simulink model "Wind_turbine_model_L"  (R2020a)
settings: Solver=ode45  StartTime=0.0  StopTime=10  RelTol=1e-3
model workspace (MAT data in the model file):
  Tw = Simulink.Parameter
  Tw.DataType = 'auto'
  Tw.Dimensions = [0 0]
undefined symbols (not defined in the file): a1, a2, a3, a4, a5, a6, a7, a8, Ad, D, denp, dent, DiscIntNeverNeededParam, f, Fs, fsw, J, ki_id, ki_n, Kopt, kp_id, kp_n, Lm, Lr, Ls, Lsi, N, nump, numt, p, Ps, Rr, Rs, sigbuilder_block, sigma, Tem, Tgd_max, Tie, Tiu, Tix, Tpe, Tpu, Tpx, Ts, Vbus, Vs, WT_Params, X, Y, Z
libraries: fl_lib x18, nesl_utility x10, sm_lib x9, powerlib x8, sdl_lib x3, powerlib_meascontrol x1, simulink x1, Yaw_Actuation_Lib x1
settings Model: Creator=param  LastModifiedBy=param

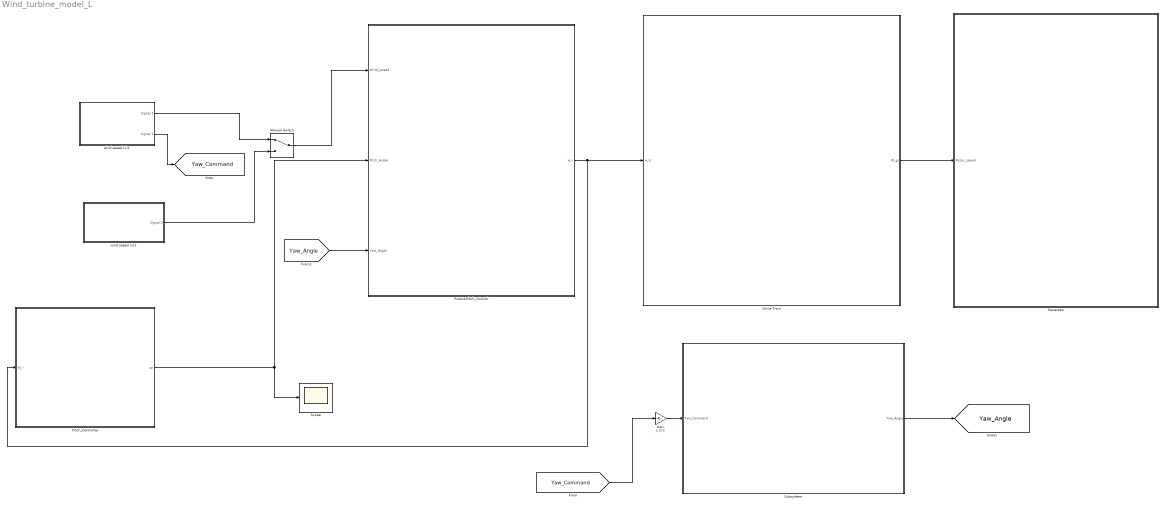
== system Wind_turbine_model_L ==
  Drive Train : Subsystem
  Gain : Gain  Gain=0.075
  Generator : Subsystem
  Manual Switch : ManualSwitch
  Pitch_Controller : Subsystem
  Rotor&Pitch_Control : Subsystem
  Scope : Scope
  Subsystem : Subsystem
  wind speed (v)1 : Subsystem  Tag=STV Subsys  LoadFcn=sigbuilder_block('load');  StartFcn=sigbuilder_block('start');  StopFcn=sigbuilder_block('stop');  ClipboardFcn=sigbuilder_block('clipboard');  mask(Sigbuilder block){tuvar=[0:10]}
      mask help: Simulink:masks:SigbuilderBlock_MD
      mask init:
      | if ~strcmp(get_param(bdroot(gcbh),'SimulationStatus'),'stopped') tuvar = sigbuilder_block('maskInit'); end
      settings: CopyFcn=sigbuilder_block('copy');  DeleteFcn=sigbuilder_block('delete');  ModelCloseFcn=sigbuilder_block('modelClose');  PreSaveFcn=sigbuilder_block('preSave');  PauseFcn=sigbuilder_block('pause');  ContinueFcn=sigbuilder_block('continue');  NameChangeFcn=sigbuilder_block('namechange');  OpenFcn=sigbuilder_block('open',[6 0 1012.5 477.75 ]);  CloseFcn=sigbuilder_block('close');
      mask Display: plot(0, 0, 100, 100,[2, 2, 32, 32, 2], [68, 8, 8, 68, 68],[32, 2], [38, 38], [32, 19, 2],[53, 60, 44], [32, 17, 17, 2],[16, 16, 31, 31]);txt = getActiveGroup(gcbh);text(2, 100, txt,'verticalAlignment', 'top');
  wind speed (v)2 : Subsystem  Tag=STV Subsys  LoadFcn=sigbuilder_block('load');  StartFcn=sigbuilder_block('start');  StopFcn=sigbuilder_block('stop');  ClipboardFcn=sigbuilder_block('clipboard');  mask(Sigbuilder block){tuvar=[0:10]}
      mask help: Simulink:masks:SigbuilderBlock_MD
      mask init:
      | if ~strcmp(get_param(bdroot(gcbh),'SimulationStatus'),'stopped') tuvar = sigbuilder_block('maskInit'); end
      settings: CopyFcn=sigbuilder_block('copy');  DeleteFcn=sigbuilder_block('delete');  ModelCloseFcn=sigbuilder_block('modelClose');  PreSaveFcn=sigbuilder_block('preSave');  PauseFcn=sigbuilder_block('pause');  ContinueFcn=sigbuilder_block('continue');  NameChangeFcn=sigbuilder_block('namechange');  OpenFcn=sigbuilder_block('open',[289.8 114 442.2 307.8 ]);  CloseFcn=sigbuilder_block('close');
      mask Display: plot(0, 0, 100, 100,[2, 2, 32, 32, 2], [68, 8, 8, 68, 68],[32, 2], [38, 38], [32, 19, 2],[53, 60, 44], [32, 17, 17, 2],[16, 16, 31, 31]);txt = getActiveGroup(gcbh);text(2, 100, txt,'verticalAlignment', 'top');
  tag scope: Yaw_Angle=global, Yaw_Command=global
  wires:
  Drive Train/1(W_gr) -> Generator/1(Rotor_speed)
  Rotor&Pitch_Control/1(w_r) -> Drive Train/1(w_tr), Pitch_Controller/1(W_r)
  Pitch_Controller/1(up) -> Scope/1, Rotor&Pitch_Control/2(Pitch_Angle)
  wind speed (v)2/1(Signal 2) -> Manual Switch/2
  Manual Switch/1 -> Rotor&Pitch_Control/1(Wind_Speed)
  wind speed (v)1/1(Signal 2) -> Manual Switch/1
  wind speed (v)1/2(Signal 1) -> [Yaw_Command]
  [Yaw_Command] -> Gain/1
  Subsystem/1(Yaw_Angle) -> [Yaw_Angle]
  [Yaw_Angle] -> Rotor&Pitch_Control/3(Yaw_Angle)
  Gain/1 -> Subsystem/1(Yaw_Command)

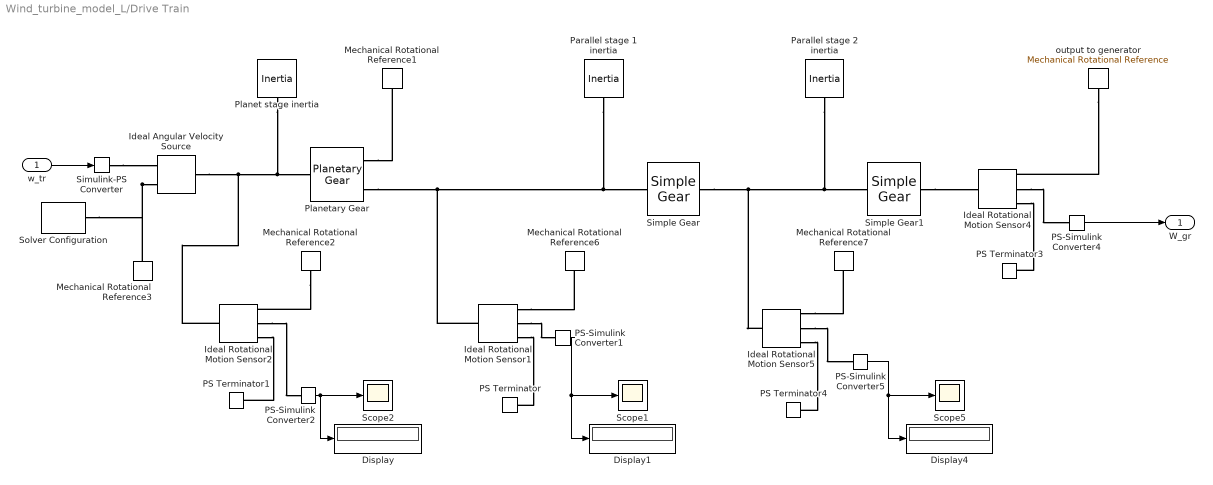
== system Wind_turbine_model_L/Drive Train ==
  w_tr : Inport
  Display : Display
  Display1 : Display
  Display4 : Display
  Ideal Angular Velocity Source : fl_lib/Mechanical/Mechanical Sources/Ideal Angular Velocity Source
  Ideal Rotational Motion Sensor{1..2,4..5} (4 alike) : fl_lib/Mechanical/Mechanical Sensors/Ideal Rotational Motion Sensor  wrap_angle=simscape.enum.onoff.off  offset=0 rad
  Mechanical Rotational Reference{1..3,6..7} (5 alike) : fl_lib/Mechanical/Rotational Elements/Mechanical Rotational Reference
  PS Terminator{,1,3..4} (4 alike) : fl_lib/Physical Signals/Sinks/PS Terminator
  PS-Simulink Converter{1..2,4..5} (4 alike) : nesl_utility/PS-Simulink Converter  PhysicalDomain=network_engine_domain  SubClassName=ps_output  LeftPortType=input  RightPortType=output  PseudoPeriodic=off  Frequencies=[]  Unit=inherit  AffineConversion=off
  Parallel stage 1 inertia : fl_lib/Mechanical/Rotational Elements/Inertia  inertia=100 kg*m^2  w_specify=off  w_priority=High  w=0 rad/s  w_nominal_specify=off  w_nominal_unit=rad/s  w_nominal_value=1  t_specify=off  t_priority=None  t=0 N*m  t_nominal_specify=off  t_nominal_unit=N*m  t_nominal_value=1
  Parallel stage 2 inertia : fl_lib/Mechanical/Rotational Elements/Inertia  inertia=100 kg*m^2  w_specify=off  w_priority=High  w=0 rad/s  w_nominal_specify=off  w_nominal_unit=rad/s  w_nominal_value=1  t_specify=off  t_priority=None  t=0 N*m  t_nominal_specify=off  t_nominal_unit=N*m  t_nominal_value=1
  Planet stage inertia : fl_lib/Mechanical/Rotational Elements/Inertia  inertia=100 kg*m^2  w_specify=off  w_priority=High  w=0 rad/s  w_nominal_specify=off  w_nominal_unit=rad/s  w_nominal_value=1  t_specify=off  t_priority=None  t=0 N*m  t_nominal_specify=off  t_nominal_unit=N*m  t_nominal_value=1
  Planetary Gear : sdl_lib/Gears/Planetary Gear  rs_ratio=7  friction_model=sdl.enum.gear_friction.none  mu_visc=[0, 0] N*m/(rad/s)  efficiency=[.96, .98]  temperature_TLU=[280, 300, 320] K  efficiency_sp_TLU=[.95, .9, .85]  efficiency_rp_TLU=[.95, .9, .85]  pwr_thr=[.001, .001] W  thermal_mass=50 J/K  T_init=300 K  model_inertia=simscape.enum.onoff.off  planet_inertia=100 kg*m^2
      settings: SourceProductBaseCode=LD
  Scope1 : Scope
  Scope2 : Scope
  Scope5 : Scope
  Simple Gear : sdl_lib/Gears/Simple Gear  ratio=1/4.5  rotation_direction=2  friction_model=sdl.enum.gear_efficiencies_load.off  T_noload=0.1 N*m  T_nom=5 N*m  efficiency_nom=0.8  efficiency=0.8  mu_visc=[0, 0] N*m/(rad/s)  w_thr=0.01 rad/s  pwr_thr=0.001 W  enable_faults=simscape.enum.onoff.off  efficiency_fault=0.05  external_fault=simscape.enum.onoff.off  temporal_fault=simscape.enum.onoff.off  fault_time=5 s  fault_angles=pi / 12 rad  report_fault=1  temperature_TLU=[280, 300, 320] K  load_TLU=[1, 5, 10] N*m  efficiency_TLU=[.95, .9, .85]  efficiency_TLU2=[.85, .8, .75; .95, .9, .85; .85, .8, .7]  thermal_mass=50 J/K  T_init=300 K
  Simple Gear1 : sdl_lib/Gears/Simple Gear  ratio=1/3.15  rotation_direction=2  friction_model=sdl.enum.gear_efficiencies_load.off  T_noload=0.1 N*m  T_nom=5 N*m  efficiency_nom=0.8  efficiency=0.8  mu_visc=[0, 0] N*m/(rad/s)  w_thr=0.01 rad/s  pwr_thr=0.001 W  enable_faults=simscape.enum.onoff.off  efficiency_fault=0.05  external_fault=simscape.enum.onoff.off  temporal_fault=simscape.enum.onoff.off  fault_time=5 s  fault_angles=pi / 12 rad  report_fault=1  temperature_TLU=[280, 300, 320] K  load_TLU=[1, 5, 10] N*m  efficiency_TLU=[.95, .9, .85]  efficiency_TLU2=[.85, .8, .75; .95, .9, .85; .85, .8, .7]  thermal_mass=50 J/K  T_init=300 K
  Simulink-PS Converter : nesl_utility/Simulink-PS Converter  PhysicalDomain=network_engine_domain  SubClassName=ps_input  LeftPortType=input  RightPortType=output  PseudoPeriodic=off  Frequencies=[]  NoiseDistribution=none  NoiseParameters=[]  Unit=1  AffineConversion=off  FilteringAndDerivatives=filter  SimscapeFilterOrder=2  InputFilterTimeConstant=0.001  UdotUserProvided=0
  Solver Configuration : nesl_utility/Solver Configuration  PhysicalDomain=network_engine_domain  SubClassName=solver  LeftPortType=input  RightPortType=generic  Tones=[]  Harmonics=[]  SimulateNoise=off  Profile=off  UseLocalSampling=off  EnableSwitchedLinearOptims=on  FrequencyDomain=off  UseCCode=off  RelTol=0.001  AbsTol=1e-06  MinStep=1e-09  ToWorkspace=off  RevertToSquareIcSolve=off  NumHomotopyIterations=100  PhasorMode=off  PhasorModeNumHarmonics=1  DoDC=off  ResidualTolerance=1e-09  UseLocalSolver=off  LocalSolverChoice=NE_BACKWARD_EULER_ADVANCER  LocalSolverSampleTime=0.001  DoFixedCost=off  MaxNonlinIter=3  MaxModeIter=2  LinearAlgebra=auto  EquationFormulation=NE_TIME_EF  DelaysMemoryBudget=1024  AutomaticFiltering=on  FilteringTimeConstant=0.001  PartitionStorageMethod=AS_NEEDED  PartitionMemoryBudget=1024  PartitionMethod=ROBUST
  output to generator : fl_lib/Mechanical/Rotational Elements/Mechanical Rotational Reference
  W_gr : Outport
  wires:
  PS-Simulink Converter1/1 -> Scope1/1, Display1/1
  PS-Simulink Converter2/1 -> Display/1, Scope2/1
  PS-Simulink Converter5/1 -> Display4/1, Scope5/1
  PS-Simulink Converter4/1 -> W_gr/1
  w_tr/1 -> Simulink-PS Converter/1
  connections:
  Ideal Angular Velocity Source/LConn1 -- Ideal Rotational Motion Sensor2/LConn1 -- Planet stage inertia/LConn1 -- Planetary Gear/LConn1
  Planetary Gear/RConn1 -- Mechanical Rotational Reference1/LConn1
  Ideal Angular Velocity Source/RConn2 -- Mechanical Rotational Reference3/LConn1 -- Solver Configuration/RConn1
  Ideal Rotational Motion Sensor1/RConn2 -- PS-Simulink Converter1/LConn1
  Ideal Rotational Motion Sensor5/RConn3 -- PS Terminator4/LConn1
  Planetary Gear/RConn2 -- Ideal Rotational Motion Sensor1/LConn1 -- Simple Gear/LConn1 -- Parallel stage 1 inertia/LConn1
  Ideal Rotational Motion Sensor1/RConn1 -- Mechanical Rotational Reference6/LConn1
  Mechanical Rotational Reference2/LConn1 -- Ideal Rotational Motion Sensor2/RConn1
  Ideal Rotational Motion Sensor4/RConn2 -- PS-Simulink Converter4/LConn1
  Ideal Rotational Motion Sensor5/RConn2 -- PS-Simulink Converter5/LConn1
  Ideal Rotational Motion Sensor2/RConn3 -- PS Terminator1/LConn1
  Simple Gear1/RConn1 -- Ideal Rotational Motion Sensor4/LConn1
  Simple Gear/RConn1 -- Ideal Rotational Motion Sensor5/LConn1 -- Parallel stage 2 inertia/LConn1 -- Simple Gear1/LConn1
  Ideal Rotational Motion Sensor4/RConn3 -- PS Terminator3/LConn1
  Ideal Rotational Motion Sensor5/RConn1 -- Mechanical Rotational Reference7/LConn1
  Ideal Rotational Motion Sensor2/RConn2 -- PS-Simulink Converter2/LConn1
  output to generator/LConn1 -- Ideal Rotational Motion Sensor4/RConn1
  Ideal Rotational Motion Sensor1/RConn3 -- PS Terminator/LConn1
  Simulink-PS Converter/RConn1 -- Ideal Angular Velocity Source/RConn1

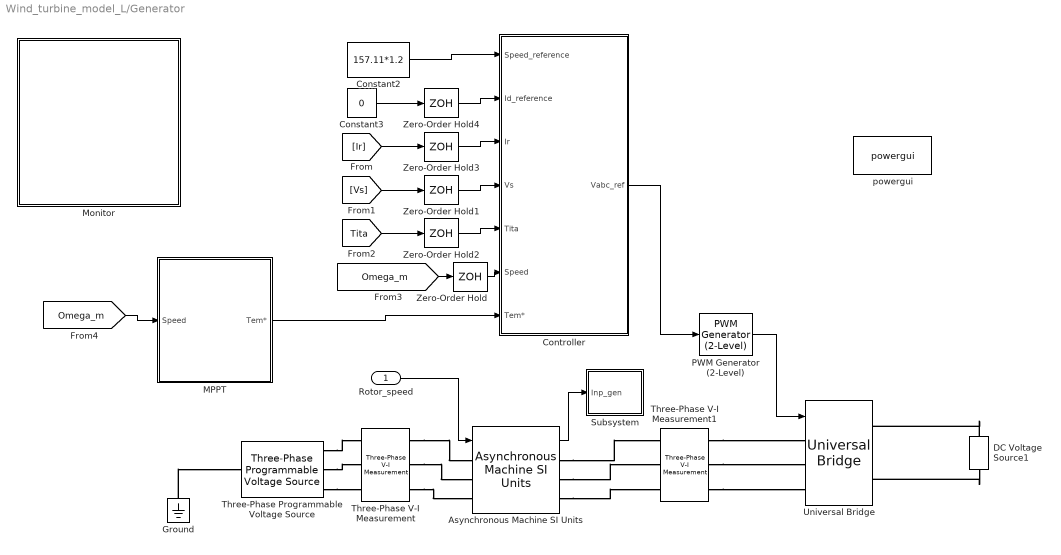
== system Wind_turbine_model_L/Generator ==
  Rotor_speed : Inport
  Asynchronous Machine SI Units : powerlib/Machines/Asynchronous Machine SI Units  RotorType=Wound  PresetModel=No  MechanicalLoad=Speed w  ShowDetailedParameters=on  ReferenceFrame=Rotor  Units=SI  MeasurementBus=off  NominalParameters=[Ps Vs f]  Stator=[Rs, Lsi]  Rotor=[Rr, Lsi]  Cage1=[0.4155 0.002066]  Cage2=[0.4168 0.0003495]  Lm=Lm  Mechanical=[J D 2]  PolePairs=2  InitialConditions=[1 0 0 0 0 0 0 0]  SimulateSaturation=off  Saturation=[14.03593122, 27.81365428, 53.79336849, 72.68890987, 97.98006896, 148.6815601, 215.7428561, 302.9841135, 428.7778367 ; 230, 322, 414, 460, 506, 552, 598, 644, 690]  LoadFlowParameters=1492000  TsPowergui=0  TsBlock=-1  IterativeModel=Trapezoidal non iterative  IterativeDiscreteModel=Trapezoidal non iterative  Pmec=1.492e+006
  Constant2 : Constant  Value=157.11*1.2
  Constant3 : Constant  Value=0
  Controller : Subsystem
  DC Voltage Source1 : powerlib/Electrical Sources/DC Voltage Source  Amplitude=Vbus  Measurements=None
  Ground : powerlib/Elements/Ground  LConnTagsString=a
  MPPT : Subsystem
  Monitor : Subsystem
  PWM Generator (2-Level) : powerlib_meascontrol/Pulse & Signal Generators/PWM Generator (2-Level)  ModulatorType=Three-phase bridge (6 pulses)  ModulatorMode=Unsynchronized  Fc=fsw  Pc=90  nF=27  MinMax="[ -1  1 ]"  SamplingTechnique=Symmetrical regular (single edge)  ModulatingSignals=off  m=0.8  Freq=60  Phase=0  Ts=0  ShowCarrierOutport=off
  Subsystem : Subsystem
  Three-Phase Programmable Voltage Source : powerlib/Electrical Sources/Three-Phase Programmable Voltage Source  PositiveSequence=[Vs 0 f]  VariationEntity=None  VariationType=Table of time-amplitude pairs  VariationTypeAlt=Step  VariationStep=0.5  VariationRate=10  VariationMagnitude=0.3  VariationFrequency=2  VariationTiming=[1 2]  VariationPhaseA=off  Amplitudes=[1 0.8 1.2 1.0]  TimeValues=[0 0.1 0.15 0.2]  HarmonicGeneration=off  HarmonicA=[3 0.2 -25 0]  HarmonicB=[2 0.15 35 2]  Timing="[0.05  3]"  BusType=swing  Pref=0  Qref=0  Qmin=-inf  Qmax=inf
  Three-Phase V-I Measurement : powerlib/Measurements/Three-Phase V-I Measurement  VoltageMeasurement=phase-to-ground  SetLabelV=on  LabelV=Vs  Vpu=on  VpuLL=off  CurrentMeasurement=yes  SetLabelI=on  LabelI=Is  Ipu=off  Pbase=100e6  Vbase=500e3  OutputType=Complex  PhasorSimulation=off  PSBequivalent=0
  Three-Phase V-I Measurement1 : powerlib/Measurements/Three-Phase V-I Measurement  VoltageMeasurement=no  SetLabelV=off  LabelV=Vr  Vpu=off  VpuLL=off  CurrentMeasurement=yes  SetLabelI=on  LabelI=Ir  Ipu=off  Pbase=100e6  Vbase=500e3  OutputType=Complex  PhasorSimulation=off  PSBequivalent=0
  Universal Bridge : powerlib/Power Electronics/Universal Bridge  Arms=3  SnubberResistance=1e5  SnubberCapacitance=inf  Device=Ideal Switches  Ron=1e-3  Lon=0  ForwardVoltages="[  0  0  ]"  ForwardVoltage=0  GTOparameters=[ 10e-6 , 20e-6 ]  IGBTparameters=[ 1e-6 , 2e-6 ]  Measurements=None  Measurements_2=None  converterType=Rectifier
  Zero-Order Hold{,1..4} (5 alike) : ZeroOrderHold  SampleTime=1/fsw
  powergui : powerlib/powergui  Priority=1  SimulationMode=Discrete  SampleTime=Ts  frequency=60  Iterations=50  frequencyindice=50  Pbase=100e6  ErrMax=1e-4  UnitsV=kV  UnitsW=MW  buscounter=0  FunctionMessages=off  echomessages=off  EnableUseOfTLC=off  CurrentSourceSwitches=off  DisableSnubberDevices=off  DisableRonSwitches=off  DisableVfSwitches=off  DisplayEquations=off  AutomaticDiscreteSolvers=off  SolverType=Tustin/Backward Euler (TBE)  Interpol=off  ExternalGateDelay=off  methode=off  Ts=100  x0status=blocks  SPID=on  SwTol=0  HookPort=off  NonlinearTolerance=1e-4  nMaxIteration=100  ContinueOnMaxIteration=off  RestoreLinks=warning  ResistiveCurrentMeasurement=off  Frange=[0:2:500]  Ylog=off  Xlog=on  ShowGrid=off  save=off  variable=ZData  structure=0  ZoomFFT=off  StartTime=0.0  cycles=1  DisplayStyle=1  fundamental=60  FreqAxis=off  MaxFrequency=1000  frequencyindicesteady=1  RmsSteady=1  display=off
  wires:
  Zero-Order Hold2/1 -> Controller/5(Tita)
  [Tita] -> Zero-Order Hold2/1
  Zero-Order Hold/1 -> Controller/6(Speed)
  [Vs] -> Zero-Order Hold1/1
  Zero-Order Hold4/1 -> Controller/2(Id_reference)
  Zero-Order Hold1/1 -> Controller/4(Vs)
  [Ir] -> Zero-Order Hold3/1
  Asynchronous Machine SI Units/1 -> Subsystem/1(Inp_gen)
  PWM Generator (2-Level)/1 -> Universal Bridge/1
  Constant2/1 -> Controller/1(Speed_reference)
  Constant3/1 -> Zero-Order Hold4/1
  [Omega_m] -> Zero-Order Hold/1
  Zero-Order Hold3/1 -> Controller/3(Ir)
  Controller/1(Vabc_ref) -> PWM Generator (2-Level)/1
  Rotor_speed/1 -> Asynchronous Machine SI Units/1
  [Omega_m] -> MPPT/1(Speed)
  MPPT/1(Tem*) -> Controller/7(Tem*)
  connections:
  Three-Phase V-I Measurement1/LConn3 -- Universal Bridge/LConn3
  Asynchronous Machine SI Units/RConn1 -- Three-Phase V-I Measurement1/RConn1
  Three-Phase V-I Measurement/RConn1 -- Asynchronous Machine SI Units/LConn1
  DC Voltage Source1/LConn1 -- Universal Bridge/RConn2
  Three-Phase Programmable Voltage Source/RConn3 -- Three-Phase V-I Measurement/LConn3
  Three-Phase V-I Measurement1/LConn2 -- Universal Bridge/LConn2
  Three-Phase Programmable Voltage Source/RConn2 -- Three-Phase V-I Measurement/LConn2
  Three-Phase Programmable Voltage Source/RConn1 -- Three-Phase V-I Measurement/LConn1
  Three-Phase V-I Measurement1/LConn1 -- Universal Bridge/LConn1
  Three-Phase V-I Measurement/RConn2 -- Asynchronous Machine SI Units/LConn2
  Three-Phase V-I Measurement/RConn3 -- Asynchronous Machine SI Units/LConn3
  Asynchronous Machine SI Units/RConn3 -- Three-Phase V-I Measurement1/RConn3
  Ground/LConn1 -- Three-Phase Programmable Voltage Source/LConn1
  DC Voltage Source1/RConn1 -- Universal Bridge/RConn1
  Asynchronous Machine SI Units/RConn2 -- Three-Phase V-I Measurement1/RConn2

== system Wind_turbine_model_L/Pitch_Controller ==
  note: um
  note: Wref
  W_r : Inport
  Controller : Subsystem
  Reference : TransferFcn  Denominator=[1 1]
  Step : Step  Time=0  After=1.8  SampleTime=0
  Sum3 : Sum  Inputs=|+-
  up : Outport
  wires:
  W_r/1 -> Sum3/2
  Step/1 -> Controller/2(um), Reference/1
  Reference/1 -> Sum3/1, Controller/1(xm)
  Sum3/1 -> Controller/3(ey)
  Controller/1(up) -> up/1

== system Wind_turbine_model_L/Rotor&Pitch_Control ==
  Wind_Speed : Inport
  Pitch_Angle : Inport  Port=2
  Yaw_Angle : Inport  Port=3
  Abs : Abs
  Constant : Constant  Commented=on  Value=Tgd_max
  Wr Plant : Subsystem
  w_r : Outport
  wires:
  Wr Plant/1(Wr(s)) -> w_r/1
  Wind_Speed/1 -> Wr Plant/1(v(s))
  [Tem_ref] -> Abs/1
  Abs/1 -> Wr Plant/3(Tgd(s))
  Pitch_Angle/1 -> Wr Plant/2(Betad(s))
  Yaw_Angle/1 -> Wr Plant/4(Yaw_Angle)

== system Wind_turbine_model_L/Subsystem ==
  Yaw_Command : Inport
  PID Controller : simulink/Continuous/PID Controller  Controller=PID  Form=Parallel  TimeDomain=Continuous-time  UseExternalTs=off  SampleTime=-1  IntegratorMethod=Forward Euler  FilterMethod=Forward Euler  ControllerParametersSource=internal  P=2.88422427280199  I=9.43357368987043  D=0.0596373379151778  UseFilter=on  N=693.993801659791  TunerSelectOption=Transfer Function Based (PID Tuner App)  InitialConditionSource=internal  InitialConditionForIntegrator=0  InitialConditionForFilter=0  DifferentiatorICPrevScaledInput=0  ExternalReset=none  TrackingMode=off  Kt=1  LimitOutput=off  UpperSaturationLimit=inf  LowerSaturationLimit=-inf  LinearizeAsGain=on  AntiWindupMode=none  Kb=1  POutMin=[]  POutMax=[]  IOutMin=[]  IOutMax=[]  DOutMin=[]  DOutMax=[]  NOutMin=[]  NOutMax=[]  SumOutMin=[]  SumOutMax=[]  SaturationOutMin=[]  SaturationOutMax=[]  PParamMin=[]  PParamMax=[]  IParamMin=[]  IParamMax=[]  DParamMin=[]  DParamMax=[]  NParamMin=[]  NParamMax=[]  KbParamMin=[]  KbParamMax=[]  KtParamMin=[]  KtParamMax=[]  KbOutMin=[]  KbOutMax=[]  KtOutMin=[]  KtOutMax=[]  IntegratorOutMin=[]  IntegratorOutMax=[]  FilterOutMin=[]  FilterOutMax=[]  SumI1OutMin=[]  SumI1OutMax=[]  SumI2OutMin=[]  SumI2OutMax=[]  SumI3OutMin=[]  SumI3OutMax=[]  SumI4OutMin=[]  SumI4OutMax=[]  SumDOutMin=[]  SumDOutMax=[]  DifferentiatorOutMin=[]  DifferentiatorOutMax=[]  FilterDiffOutCoefMin=[]  FilterDiffOutCoefMax=[]  ReciprocalOutMin=[]  ReciprocalOutMax=[]  SumDenOutMin=[]  SumDenOutMax=[]  SumNumOutMin=[]  SumNumOutMax=[]  DivideOutMin=[]  DivideOutMax=[]  UdiffTsProdOutMin=[]  UdiffTsProdOutMax=[]  NTsProdOutMin=[]  NTsProdOutMax=[]  UintegralTsProdOutMin=[]  UintegralTsProdOutMax=[]  UngainTsProdOutMin=[]  UngainTsProdOutMax=[]  IntegratorContinuousStateAttributes=''  IntegratorStateMustResolveToSignalObject=off  IntegratorRTWStateStorageClass=Auto  FilterContinuousStateAttributes=''  FilterStateMustResolveToSignalObject=off  FilterRTWStateStorageClass=Auto  ParallelPVariant=InternalParameters  IdealPVariant=Disabled  IVariant=InternalParameters  DVariant=InternalParameters  IntegratorVariant=Continuous  SatVariant=Disabled  AWVariant=Passthrough  PCopyVariant=Disabled  TRVariant=Disabled  FdbkBlocksVariant=Forward  IdealPFdbkVariant=Disabled  SatFdbkVariant=Disabled  DerivativeFilterVariant=ContFilter  NVariant=InternalParameters  NCopyVariant=Disabled  FilterICVariant=InternalICsFilter  IntegratorICVariant=InternalICs  ExternalResetVariant=Disabled  TRSumVariant=Passthrough  SumFdbkVariant=Disabled  SumVariant=Sum_PID  TsampFilterVariant=InternalTs  TsampNgainVariant=Passthrough  TsampIntegralVariant=Passthrough
  Solver Configuration : nesl_utility/Solver Configuration  Commented=on  PhysicalDomain=network_engine_domain  SubClassName=solver  LeftPortType=input  RightPortType=generic  Tones=[]  Harmonics=[]  SimulateNoise=off  Profile=off  UseLocalSampling=off  EnableSwitchedLinearOptims=on  FrequencyDomain=off  UseCCode=off  RelTol=0.001  AbsTol=1e-06  MinStep=1e-09  ToWorkspace=off  RevertToSquareIcSolve=off  NumHomotopyIterations=100  PhasorMode=off  PhasorModeNumHarmonics=1  DoDC=off  ResidualTolerance=1e-09  UseLocalSolver=off  LocalSolverChoice=NE_BACKWARD_EULER_ADVANCER  LocalSolverSampleTime=0.001  DoFixedCost=off  MaxNonlinIter=3  MaxModeIter=2  LinearAlgebra=auto  EquationFormulation=NE_TIME_EF  DelaysMemoryBudget=1024  AutomaticFiltering=on  FilteringTimeConstant=0.001  PartitionStorageMethod=AS_NEEDED  PartitionMemoryBudget=1024  PartitionMethod=ROBUST
  Subsystem : Subsystem  Commented=on
  Sum : Sum  Inputs=|+-
  Transfer Fcn : TransferFcn  Numerator=[35]  Denominator=[1 18 35]
  Yaw System : Subsystem  Tag=CustomStyle  Commented=on  Variant=on  VariantControlMode=Label  LabelModeActiveChoice=Ideal_Actuator
      settings: AttributesFormatString=%<ActiveVariant>
      mask Display:
      | blk = find_system(gcbh, 'SearchDepth', 1, 'Parent', gcb, 'VariantObject', get_param(gcb,'activevariant'));
      | eval(get_param(blk, 'MaskDisplay'));
  Yaw_Angle : Outport
  wires:
  Transfer Fcn/1 -> Sum/2, Yaw_Angle/1
  PID Controller/1 -> Transfer Fcn/1
  Yaw_Command/1 -> Sum/1
  Sum/1 -> PID Controller/1
  connections:
  Yaw System/LConn1 -- Subsystem/LConn1
  Solver Configuration/RConn1 -- Subsystem/RConn1

== system Wind_turbine_model_L/wind speed (v)1 ==
  Demux : Demux  Tag=STV Demux  Outputs=2
      settings: DisplayOption=none
  FromWs : FromWorkspace  Tag=STV FromWs  VariableName=tuvar
      SigBuilderData=|
      | common.afterFinalStr = 'Extrapolate'
      | common.sampleTime = 0
      | dataSet(1).timeRange = [0 120]
      | dataSet(1).name = 'Group 1'
      | dataSet(2).timeRange = [0 10]
      | dataSet(2).name = 'Group 2'
      | sbobj.Groups(1).Name = 'Group 1'
      | sbobj.Groups(1).Signals(1).Name = 'Signal 2'
      | sbobj.Groups(1).Signals(1).XData = [0 0.1 0.2 0.3 0.4 0.5 0.6 0.7 0.8 0.9 1 1.1 ... (1201 elements, 1x1201)]
      | sbobj.Groups(1).Signals(1).YData = [15.5376671395 16.8338850146 12.741153139 15.8621733204 15.3187652399 13.6923117037 14.5664079777 15.3426244665 18.5783969397 17.7694370299 13.6501130598 18.0349234663 ... (1201 elements, 1x1201)]
      | sbobj.Groups(1).Signals(2).Name = 'Signal 1'
      | sbobj.Groups(1).Signals(2).XData = [0 10 120]
      | sbobj.Groups(1).Signals(2).YData = [6.19231170369 7.06640797769 7.06640797769]
      | sbobj.Groups(1).TimeRange = [0 120]
      | sbobj.Groups(2).Name = 'Group 2'
      | sbobj.Groups(2).Signals(1).Name = 'Signal 2'
      | sbobj.Groups(2).Signals(1).XData = [0 2 4 6 8 10]
      | sbobj.Groups(2).Signals(1).YData = [15.2036737857 20.7 12.9 20.8 19.2 19.2]
      | sbobj.Groups(2).Signals(2).Name = 'Signal 1'
      | sbobj.Groups(2).Signals(2).XData = [0 2 4 6 8 10]
      | sbobj.Groups(2).Signals(2).YData = [8.65011305984 13.0349234663 10.7254042249 9.93694512681 10.7147429038 9.7950339417]
  Signal 2 : Outport  Tag=STV Outport
  Signal 1 : Outport  Tag=STV Outport  Port=2
  wires:
  Demux/1 -> Signal 2/1
  FromWs/1 -> Demux/1
  Demux/2 -> Signal 1/1

== system Wind_turbine_model_L/wind speed (v)2 ==
  Demux : Demux  Tag=STV Demux  Outputs=1
      settings: DisplayOption=none
  FromWs : FromWorkspace  Tag=STV FromWs  VariableName=tuvar
      SigBuilderData=|
      | common.afterFinalStr = 'Extrapolate'
      | common.sampleTime = 0
      | dataSet(1).timeRange = [0 120]
      | dataSet(1).name = 'Group 1'
      | dataSet(2).timeRange = [0 120]
      | dataSet(2).name = 'Group 2'
      | sbobj.Groups(1).Name = 'Group 1'
      | sbobj.Groups(1).Signals.Name = 'Signal 2'
      | sbobj.Groups(1).Signals.XData = [0 0.1 0.2 0.3 0.4 0.5 0.6 0.7 0.8 0.9 1 1.1 ... (1201 elements, 1x1201)]
      | sbobj.Groups(1).Signals.YData = [15.5376671395 16.8338850146 12.741153139 15.8621733204 15.3187652399 13.6923117037 14.5664079777 15.3426244665 18.5783969397 17.7694370299 13.6501130598 18.0349234663 ... (1201 elements, 1x1201)]
      | sbobj.Groups(1).TimeRange = [0 120]
      | sbobj.Groups(2).Name = 'Group 2'
      | sbobj.Groups(2).Signals.Name = 'Signal 2'
      | sbobj.Groups(2).Signals.XData = [0 0.1 0.2 0.3 0.4 0.5 0.6 0.7 0.8 0.9 1 1.1 ... (1201 elements, 1x1201)]
      | sbobj.Groups(2).Signals.YData = [4.38462340739 6.13281595539 7.68524893308 14.1567938795 12.5388740598 4.30022611969 13.0698469327 8.45080844989 6.87389025362 8.42948580765 6.5900678834 6.75171130357 ... (1201 elements, 1x1201)]
      | sbobj.Groups(2).TimeRange = [0 120]
  Signal 2 : Outport  Tag=STV Outport
  wires:
  Demux/1 -> Signal 2/1
  FromWs/1 -> Demux/1

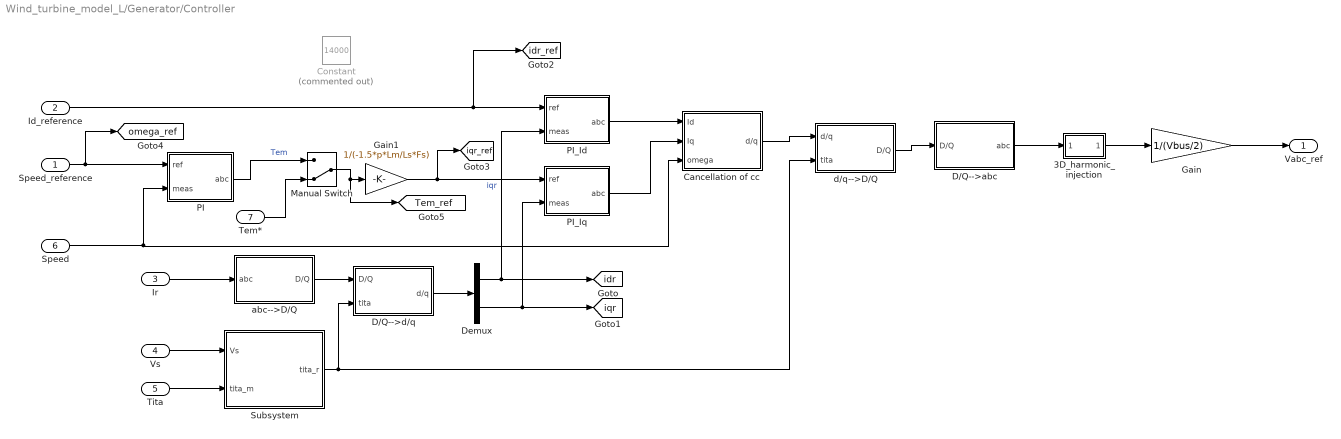
== system Wind_turbine_model_L/Generator/Controller ==
  Speed_reference : Inport
  Id_reference : Inport  Port=2
  Ir : Inport  Port=3
  Vs : Inport  Port=4
  Tita : Inport  Port=5
  Speed : Inport  Port=6
  Tem* : Inport  Port=7
  3D_harmonic_injection : Subsystem
  Cancellation of cc : Subsystem
  Constant : Constant  Commented=on  Value=14000
  D/Q-->abc : Subsystem
  D/Q-->d/q : Subsystem
  Demux : Demux  Outputs=2
  Gain : Gain  Gain=1/(Vbus/2)
  Gain1 : Gain  Gain=1/(-1.5*p*Lm/Ls*Fs)
  Manual Switch : ManualSwitch  CurrentSetting=0
  PI : Subsystem
  PI_Id : Subsystem
  PI_Iq : Subsystem
  Subsystem : Subsystem
  abc-->D/Q : Subsystem
  d/q-->D/Q : Subsystem
  Vabc_ref : Outport
  tag scope: Tem_ref=global, idr=global, idr_ref=global, iqr=global, iqr_ref=global, omega_ref=global
  wires:
  Id_reference/1 -> PI_Id/1(ref), [idr_ref]
  Gain1/1 -> PI_Iq/1(ref), [iqr_ref]  "iqr"
  Speed_reference/1 -> PI/1(ref), [omega_ref]
  Cancellation of cc/1(d/q) -> d/q-->D/Q/1(d/q)
  PI_Iq/1(abc) -> Cancellation of cc/2(Iq)
  PI_Id/1(abc) -> Cancellation of cc/1(Id)
  Demux/2 -> [iqr], PI_Iq/2(meas)
  Demux/1 -> [idr], PI_Id/2(meas)
  D/Q-->d/q/1(d/q) -> Demux/1
  Speed/1 -> Cancellation of cc/3(omega), PI/2(meas)
  Tita/1 -> Subsystem/2(tita_m)
  Vs/1 -> Subsystem/1(Vs)
  Subsystem/1(tita_r) -> D/Q-->d/q/2(tita), d/q-->D/Q/2(tita)
  3D_harmonic_injection/1(out1) -> Gain/1
  Ir/1 -> abc-->D/Q/1(abc)
  abc-->D/Q/1(D/Q) -> D/Q-->d/q/1(D/Q)
  d/q-->D/Q/1(D/Q) -> D/Q-->abc/1(D/Q)
  Gain/1 -> Vabc_ref/1
  D/Q-->abc/1(abc) -> 3D_harmonic_injection/1(ln1)
  PI/1(abc) -> Manual Switch/1  "Tem"
  Manual Switch/1 -> [Tem_ref], Gain1/1
  Tem*/1 -> Manual Switch/2

== system Wind_turbine_model_L/Generator/MPPT ==
  Speed : Inport
  Gain : Gain  Gain=1/N
  Gain1 : Gain  Gain=-Kopt
  Gain2 : Gain  Gain=1/N
  Square : Math  Operator=square  SaturateOnIntegerOverflow=on
  Tem* : Outport
  wires:
  Speed/1 -> Gain/1
  Gain/1 -> Square/1
  Square/1 -> Gain1/1
  Gain1/1 -> Gain2/1
  Gain2/1 -> Tem*/1

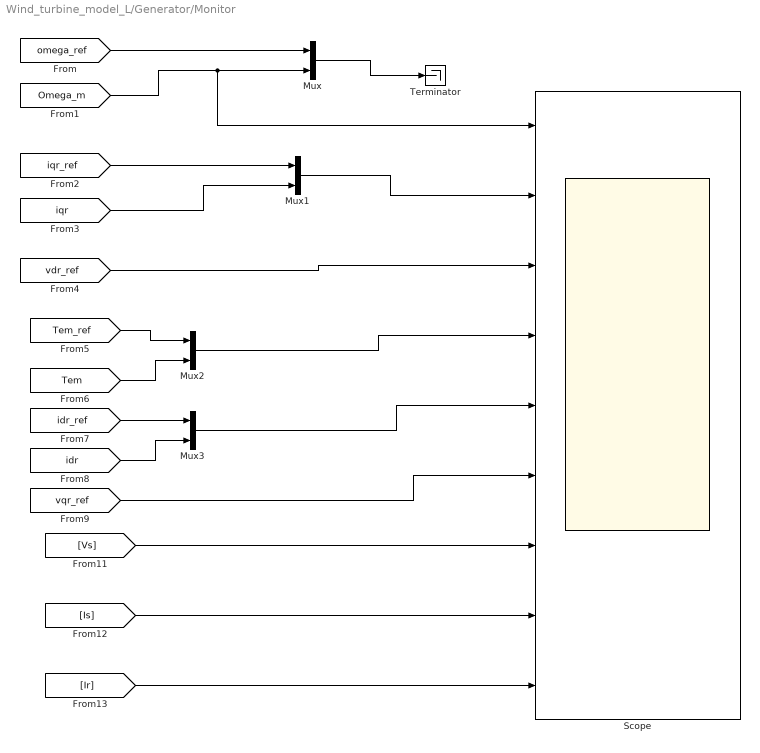
== system Wind_turbine_model_L/Generator/Monitor ==
  Mux{,1..3} (4 alike) : Mux  Inputs=2
  Scope : Scope  NumInputPorts=9
  Terminator : Terminator
  wires:
  [Ir] -> Scope/9
  [Is] -> Scope/8
  [Vs] -> Scope/7
  [vqr_ref] -> Scope/6
  Mux3/1 -> Scope/5
  Mux2/1 -> Scope/4
  [vdr_ref] -> Scope/3
  Mux1/1 -> Scope/2
  [idr] -> Mux3/2
  [idr_ref] -> Mux3/1
  [Tem] -> Mux2/2
  [Tem_ref] -> Mux2/1
  [iqr] -> Mux1/2
  [iqr_ref] -> Mux1/1
  [Omega_m] -> Scope/1, Mux/2
  [omega_ref] -> Mux/1
  Mux/1 -> Terminator/1

== system Wind_turbine_model_L/Generator/Subsystem ==
  Inp_gen : Inport
  Bus Selector : BusSelector  OutputSignals=Mechanical.Rotor angle thetam (rad),Mechanical.Rotor speed (wm),Mechanical.Electromagnetic torque Te (N*m)
  tag scope: Omega_m=global, Tem=global, Tita=global
  wires:
  Bus Selector/3 -> [Tem]  "<Electromagnetic torque Te (N*m)>"
  Bus Selector/2 -> [Omega_m]  "<Rotor speed (wm)>"
  Bus Selector/1 -> [Tita]  "<Rotor angle thetam (rad)>"
  Inp_gen/1 -> Bus Selector/1

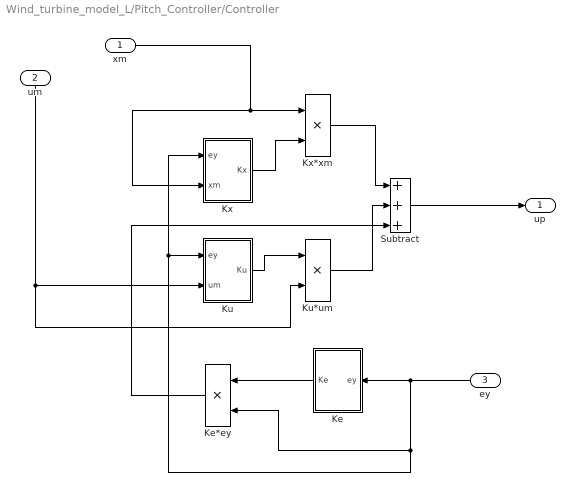
== system Wind_turbine_model_L/Pitch_Controller/Controller ==
  xm : Inport
  um : Inport  Port=2
  ey : Inport  Port=3
  Ke : Subsystem
  Ke*ey : Product
  Ku : Subsystem
  Ku*um : Product
  Kx : Subsystem
  Kx*xm : Product
  Subtract : Sum  Inputs=+++
  up : Outport
  wires:
  Kx/1(Kx) -> Kx*xm/2
  Ke/1(Ke) -> Ke*ey/1
  Ku*um/1 -> Subtract/2
  Kx*xm/1 -> Subtract/1
  xm/1 -> Kx*xm/1, Kx/2(xm)
  ey/1 -> Kx/1(ey), Ku/1(ey), Ke*ey/2, Ke/1(ey)
  Ku/1(Ku) -> Ku*um/1
  Ke*ey/1 -> Subtract/3
  um/1 -> Ku/2(um), Ku*um/2
  Subtract/1 -> up/1

== system Wind_turbine_model_L/Rotor&Pitch_Control/Wr Plant ==
  note: yp
  note: Tg(s)
  v(s) : Inport
  Betad(s) : Inport  Port=2
  Tgd(s) : Inport  Port=3
  Yaw_Angle : Inport  Port=4
  GTg(s) : TransferFcn  Numerator=numt  Denominator=dent
  GTr(s) : TransferFcn  Numerator=nump  Denominator=denp
  Sum : Sum
  Wind Turbine : Subsystem  AncestorBlock=re_lib/Wind Generation/Wind Turbine  DialogController=POWERSYS.PowerSysDialog  mask(Wind Turbine){Pnom=2e6, Pelec_base=2e6/0.9, wind_base=9, P_wind_base=0.73, speed_nom=1.2, pitch_angle=10, c1_c6=[0.51763          116          0.4            5           21     0.006795], cp_nom=0.48, lambda_nom=8.1}
      mask prompts: Pnom "Nominal mechanical output power (W):"; Pelec_base "Base power of the electrical generator (VA):"; wind_base "Base wind speed (m/s):"; P_wind_base "Maximum power at base wind speed (pu of nominal mechanical power):"; speed_nom "Base rotational speed (p.u. of base generator speed):"; pitch_angle "Pitch angle beta to display wind-turbine power characteristics (beta >=0)  (deg):"
      mask help:
      | This block implements a variable pitch wind turbine model. The performance coefficient Cp of the turbine is the mechanical output power of the turbine divided by wind power and a function of wind speed, rotational speed, and pitch angle (beta). Cp reaches its maximum value at zero beta. Select the wind-turbine power characteristics display to plot the turbine characteristics at the specified pitch angle.
      |
      | The first input is the generator speed in per unit of the generator base speed. For a synchronous or asynchronous generator, the base speed is the synchronous speed. For a permanent-magnet generator, the base speed is defined as the speed producing nominal voltage at  no load. The second input is the blade pitch angle (beta) in degrees. The third input is the wind speed in m/s.
      |
      | The output is the torque applied to the generator shaft in per unit of the generator ratings.
      |
      | The turbine inertia must be added to the generator inertia.
      mask init:
      | c1=c1_c6(1);c2=c1_c6(2);c3=c1_c6(3);c4=c1_c6(4);c5=c1_c6(5);c6=c1_c6(6);
      | power_initmask();
      mask Help: helpview(psbhelp);
      mask DialogControl DisplayTurbChar Prompt: Display wind turbine power characteristics
      mask DialogControl DisplayTurbChar Callback: WindTurbinePlot(gcb)
      mask Display: disp('');
  Wr(s) : Outport
  wires:
  v(s)/1 -> Wind Turbine/3(v(s))
  Sum/1 -> Wind Turbine/1(Wr(s)), Wr(s)/1
  Tgd(s)/1 -> GTg(s)/1
  GTg(s)/1 -> Sum/2
  GTr(s)/1 -> Sum/1
  Betad(s)/1 -> Wind Turbine/2(Beta(s))
  Wind Turbine/1(Tr(s)) -> GTr(s)/1
  Yaw_Angle/1 -> Wind Turbine/4(Yaw_Angle)

== system Wind_turbine_model_L/Subsystem/Subsystem ==
  Mechanism Configuration : sm_lib/Utilities/Mechanism Configuration  UniformGravity=Constant  GravityVector=[0 0 -9.81]*0  GravityUnits=m/s^2  LinearizationDelta=0.001
  Solid : sm_lib/Body Elements/Revolved Solid  GraphicAmbientColor=[0.15 0.15 0.15 1.0]  BasedOnType=Density  CenterOfMass=[0 0 0]  CenterOfMassUnits=m  GraphicDiffuseColor=[0.8 0.8 0.8]  ExportConvexHullGeometry=off  Density=1000  DensityUnits=kg/(m^3)  DoExposeReferenceFrame=on  GraphicEmissiveColor=[0.0 0.0 0.0 1.0]  ExportEntireGeometry=off  SerializedFrames=<Frames/>  MarkerShape=Sphere  MarkerSize=10  GraphicType=FromGeometry  InertiaType=CalculateFromGeometry  Mass=1  MassUnits=kg  MomentsOfInertia=[1 1 1]  MomentsOfInertiaUnits=kg*m^2  GraphicOpacity=1.0  ProductsOfInertia=[0 0 0]  ProductsOfInertiaUnits=kg*m^2  RevolutionCrossSection=[0 -WT_Params.Tower.height/2;WT_Params.Tower.base_radius -WT_Params.Tower.height/2;WT_Params.Tower.top_radius WT_Params.Tower.height/2;0 WT_Params.Tower.height/2]  RevolutionCrossSectionUnits=m  RevolutionAngle=180  RevolutionAngleUnits=deg  RevolutionExtent=Full  GraphicShininess=75  GraphicSpecularColor=[0.5 0.5 0.5 1.0]  GraphicVisPropType=SimpleVisualProperties
  Transform TowerCtr : sm_lib/Frames and Transforms/Rigid Transform  TranslationMethod=StandardAxis  TranslationStandardOffset=WT_Params.Tower.height/2  TranslationLengthUnit=m  TranslationStandardAxis=+Z  TranslationCartesianOffset=[0 0 0]  TranslationROffset=0  TranslationROffsetUnits=m  TranslationZOffset=0  TranslationZOffsetUnits=m  TranslationThetaOffset=0  TranslationThetaOffsetUnits=deg  RotationMethod=None  RotationAngleUnits=deg  RotationStandardAxis=+Z  RotationAngle=0  RotationArbitraryAxis=[0 0 1]  FollAlignAxisA=+X  BaseAlignAxisA=+Y  FollAlignAxisB=+Y  BaseAlignAxisB=+Z  RotationSequenceAxes=FollowerAxes  RotationSequence=XYX  RotationSequenceAngles=[0 0 0]  RotationSequenceAnglesUnits=deg  RotationMatrix=[1 0 0; 0 1 0; 0 0 1]
  Transform TowerTop : sm_lib/Frames and Transforms/Rigid Transform  TranslationMethod=StandardAxis  TranslationStandardOffset=WT_Params.Tower.height/2  TranslationLengthUnit=m  TranslationStandardAxis=+Z  TranslationCartesianOffset=[0 0 0]  TranslationROffset=0  TranslationROffsetUnits=m  TranslationZOffset=0  TranslationZOffsetUnits=m  TranslationThetaOffset=0  TranslationThetaOffsetUnits=deg  RotationMethod=None  RotationAngleUnits=deg  RotationStandardAxis=+Z  RotationAngle=0  RotationArbitraryAxis=[0 0 1]  FollAlignAxisA=+X  BaseAlignAxisA=+Y  FollAlignAxisB=+Y  BaseAlignAxisB=+Z  RotationSequenceAxes=FollowerAxes  RotationSequence=XYX  RotationSequenceAngles=[0 0 0]  RotationSequenceAnglesUnits=deg  RotationMatrix=[1 0 0; 0 1 0; 0 0 1]
  World Frame : sm_lib/Frames and Transforms/World Frame
  N : PMIOPort  Side=Left
  Env : PMIOPort  Port=2  Side=Right
  connections:
  Solid/RConn1 -- Transform TowerCtr/RConn1 -- Transform TowerTop/LConn1
  Env/RConn1 -- Mechanism Configuration/RConn1 -- Transform TowerCtr/LConn1 -- World Frame/RConn1
  Transform TowerTop/RConn1 -- N/RConn1

== system Wind_turbine_model_L/Subsystem/Yaw System ==
  Ideal Actuator : Subsystem  AncestorBlock=Yaw_System_Lib/Ideal Actuator  VariantControl=Ideal_Actuator
      mask Display: image('Yaw_Ideal_Actuator_System_IMAGE.jpg');
  N : PMIOPort  Side=Right
  T : PMIOPort  Port=2  Side=Left
  YC : PMIOPort  Port=3  Side=Right

== system Wind_turbine_model_L/Generator/Controller/3D_harmonic_injection ==
  ln1 : Inport
  Gain : Gain  Gain=-0.5
  Max : MinMax  Function=max
  Min : MinMax
  Sum : Sum  Inputs=|++
  Sum1 : Sum  Inputs=|++
  out1 : Outport
  wires:
  Sum1/1 -> out1/1
  ln1/1 -> Sum1/1, Min/1, Max/1
  Gain/1 -> Sum1/2
  Max/1 -> Sum/2
  Min/1 -> Sum/1
  Sum/1 -> Gain/1

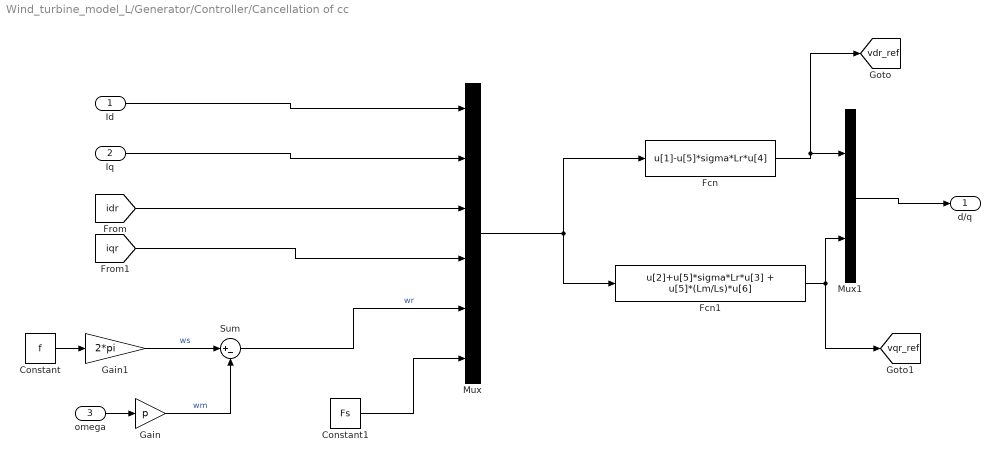
== system Wind_turbine_model_L/Generator/Controller/Cancellation of cc ==
  Id : Inport
  Iq : Inport  Port=2
  omega : Inport  Port=3
  Constant : Constant  Value=f
  Constant1 : Constant  Value=Fs
  Fcn : Fcn  Expr=u[1]-u[5]*sigma*Lr*u[4]
  Fcn1 : Fcn  Expr=u[2]+u[5]*sigma*Lr*u[3] + u[5]*(Lm/Ls)*u[6]
  Gain : Gain  Gain=p
  Gain1 : Gain  Gain=2*pi
  Mux : Mux  Inputs=6
  Mux1 : Mux  Inputs=2
  Sum : Sum  Inputs=|+-
  d/q : Outport
  tag scope: vdr_ref=global, vqr_ref=global
  wires:
  Mux1/1 -> d/q/1
  Fcn1/1 -> Mux1/2, [vqr_ref]
  Fcn/1 -> Mux1/1, [vdr_ref]
  Mux/1 -> Fcn/1, Fcn1/1
  Constant1/1 -> Mux/6
  Sum/1 -> Mux/5  "wr"
  [iqr] -> Mux/4
  [idr] -> Mux/3
  Iq/1 -> Mux/2
  Id/1 -> Mux/1
  Gain/1 -> Sum/2  "wm"
  Gain1/1 -> Sum/1  "ws"
  Constant/1 -> Gain1/1
  omega/1 -> Gain/1

== system Wind_turbine_model_L/Generator/Controller/D//Q-->abc ==
  D/Q : Inport
  Fcn : Fcn  Expr=u[1]
  Fcn1 : Fcn  Expr=-(u[1]/2) + u[2]*(sqrt(3)/2)
  Fcn2 : Fcn  Expr=-(u[1]/2) - u[2]*(sqrt(3)/2)
  Mux : Mux  Inputs=3
  abc : Outport
  wires:
  Mux/1 -> abc/1
  Fcn2/1 -> Mux/3
  Fcn1/1 -> Mux/2
  Fcn/1 -> Mux/1
  D/Q/1 -> Fcn/1, Fcn1/1, Fcn2/1

== system Wind_turbine_model_L/Generator/Controller/D//Q-->d//q ==
  D/Q : Inport
  tita : Inport  Port=2
  Fcn : Fcn  Expr=u[1]*cos(u[3])+u[2]*sin(u[3])
  Fcn1 : Fcn  Expr=-u[1]*sin(u[3]) + u[2]*cos(u[3])
  Mux : Mux  Inputs=2
  Mux1 : Mux  Inputs=2
  d/q : Outport
  wires:
  Mux1/1 -> Fcn1/1, Fcn/1
  tita/1 -> Mux1/2
  D/Q/1 -> Mux1/1
  Mux/1 -> d/q/1
  Fcn1/1 -> Mux/2
  Fcn/1 -> Mux/1

== system Wind_turbine_model_L/Generator/Controller/PI ==
  ref : Inport
  meas : Inport  Port=2
  Discrete-Time Integrator : DiscreteIntegrator  SampleTime=1/fsw  LimitOutput=on  UpperSaturationLimit=Tem  LowerSaturationLimit=-Tem  ICPrevOutput=DiscIntNeverNeededParam  ICPrevScaledInput=DiscIntNeverNeededParam
  Gain : Gain  Gain=kp_n
  Gain1 : Gain  Gain=ki_n
  Saturation : Saturate  UpperLimit=Tem  LowerLimit=-Tem
  Sum : Sum  Inputs=|+-
  Sum1 : Sum  Inputs=|++
  abc : Outport
  wires:
  Saturation/1 -> abc/1
  Discrete-Time Integrator/1 -> Sum1/2
  Sum1/1 -> Saturation/1
  Gain/1 -> Sum1/1
  Gain1/1 -> Discrete-Time Integrator/1
  Sum/1 -> Gain/1, Gain1/1
  meas/1 -> Sum/2
  ref/1 -> Sum/1

== system Wind_turbine_model_L/Generator/Controller/PI_Id ==
  ref : Inport
  meas : Inport  Port=2
  Discrete-Time Integrator : DiscreteIntegrator  SampleTime=1/fsw  LimitOutput=on  UpperSaturationLimit=Vbus/sqrt(3)  LowerSaturationLimit=-Vbus/sqrt(3)  ICPrevOutput=DiscIntNeverNeededParam  ICPrevScaledInput=DiscIntNeverNeededParam
  Gain : Gain  Gain=kp_id
  Gain1 : Gain  Gain=ki_id
  Saturation : Saturate  UpperLimit=Vbus/sqrt(3)  LowerLimit=-Vbus/sqrt(3)
  Sum : Sum  Inputs=|+-
  Sum1 : Sum  Inputs=|++
  abc : Outport
  wires:
  Saturation/1 -> abc/1
  Discrete-Time Integrator/1 -> Sum1/2
  Sum1/1 -> Saturation/1
  Gain/1 -> Sum1/1
  Gain1/1 -> Discrete-Time Integrator/1
  Sum/1 -> Gain/1, Gain1/1
  meas/1 -> Sum/2
  ref/1 -> Sum/1

== system Wind_turbine_model_L/Generator/Controller/PI_Iq ==
  ref : Inport
  meas : Inport  Port=2
  Discrete-Time Integrator : DiscreteIntegrator  SampleTime=1/fsw  LimitOutput=on  UpperSaturationLimit=Vbus/sqrt(3)  LowerSaturationLimit=-Vbus/sqrt(3)  ICPrevOutput=DiscIntNeverNeededParam  ICPrevScaledInput=DiscIntNeverNeededParam
  Gain : Gain  Gain=kp_id
  Gain1 : Gain  Gain=ki_id
  Saturation : Saturate  UpperLimit=Vbus/sqrt(3)  LowerLimit=-Vbus/sqrt(3)
  Sum : Sum  Inputs=|+-
  Sum1 : Sum  Inputs=|++
  abc : Outport
  wires:
  Saturation/1 -> abc/1
  Discrete-Time Integrator/1 -> Sum1/2
  Sum1/1 -> Saturation/1
  Gain/1 -> Sum1/1
  Gain1/1 -> Discrete-Time Integrator/1
  Sum/1 -> Gain/1, Gain1/1
  meas/1 -> Sum/2
  ref/1 -> Sum/1

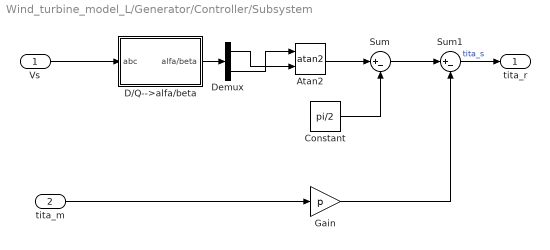
== system Wind_turbine_model_L/Generator/Controller/Subsystem ==
  Vs : Inport
  tita_m : Inport  Port=2
  Atan2 : Trigonometry  Operator=atan2
  Constant : Constant  Value=pi/2
  D/Q-->alfa/beta : Subsystem
  Demux : Demux  Outputs=2
  Gain : Gain  Gain=p
  Sum : Sum  Inputs=|+-
  Sum1 : Sum  Inputs=|+-
  tita_r : Outport
  wires:
  Gain/1 -> Sum1/2
  Sum1/1 -> tita_r/1  "tita_s"
  tita_m/1 -> Gain/1
  Sum/1 -> Sum1/1
  Constant/1 -> Sum/2
  Atan2/1 -> Sum/1
  Demux/2 -> Atan2/1
  Demux/1 -> Atan2/2
  D/Q-->alfa/beta/1(alfa/beta) -> Demux/1
  Vs/1 -> D/Q-->alfa/beta/1(abc)

== system Wind_turbine_model_L/Generator/Controller/abc-->D//Q ==
  abc : Inport
  Fcn : Fcn  Expr=2/3*(u[1]-u[2]/2-u[3]/2)
  Fcn1 : Fcn  Expr=2/3*(u[2]*(sqrt(3)/2)-u[3]*(sqrt(3)/2))
  Mux : Mux  Inputs=2
  D/Q : Outport
  wires:
  Mux/1 -> D/Q/1
  Fcn1/1 -> Mux/2
  Fcn/1 -> Mux/1
  abc/1 -> Fcn/1, Fcn1/1

== system Wind_turbine_model_L/Generator/Controller/d//q-->D//Q ==
  d/q : Inport
  tita : Inport  Port=2
  Fcn : Fcn  Expr=u[1]*cos(u[3])-u[2]*sin(u[3])
  Fcn1 : Fcn  Expr=u[1]*sin(u[3])+u[2]*cos(u[3])
  Mux : Mux  Inputs=2
  Mux1 : Mux  Inputs=2
  D/Q : Outport
  wires:
  Mux1/1 -> Fcn1/1, Fcn/1
  tita/1 -> Mux1/2
  d/q/1 -> Mux1/1
  Mux/1 -> D/Q/1
  Fcn1/1 -> Mux/2
  Fcn/1 -> Mux/1

== system Wind_turbine_model_L/Pitch_Controller/Controller/Ke ==
  ey : Inport
  Gain : Gain  Gain=Tpe
  Gain1 : Gain  Gain=Tie
  Gain2 : Gain  Gain=sigma
  Integrator : Integrator
  Product : Product
  Subtract : Sum
  Subtract1 : Sum  Inputs=+-
  Ke : Outport
  wires:
  Subtract/1 -> Ke/1
  ey/1 -> Product/2, Product/1
  Product/1 -> Gain1/1, Gain/1
  Gain/1 -> Subtract/1
  Gain1/1 -> Subtract1/1
  Subtract1/1 -> Integrator/1
  Integrator/1 -> Gain2/1, Subtract/2
  Gain2/1 -> Subtract1/2

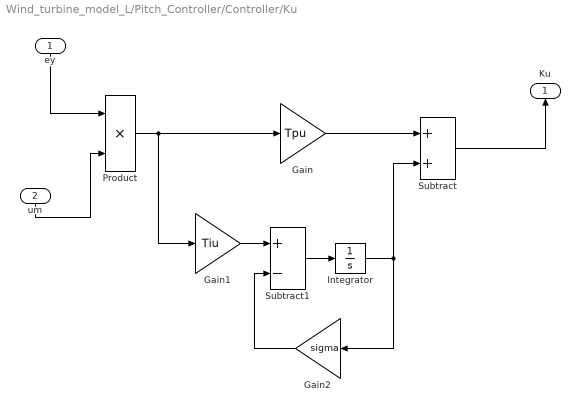
== system Wind_turbine_model_L/Pitch_Controller/Controller/Ku ==
  ey : Inport
  um : Inport  Port=2
  Gain : Gain  Gain=Tpu
  Gain1 : Gain  Gain=Tiu
  Gain2 : Gain  Gain=sigma
  Integrator : Integrator
  Product : Product
  Subtract : Sum
  Subtract1 : Sum  Inputs=+-
  Ku : Outport
  wires:
  Gain2/1 -> Subtract1/2
  Integrator/1 -> Subtract/2, Gain2/1
  Subtract1/1 -> Integrator/1
  Gain1/1 -> Subtract1/1
  Gain/1 -> Subtract/1
  Product/1 -> Gain/1, Gain1/1
  Subtract/1 -> Ku/1
  ey/1 -> Product/1
  um/1 -> Product/2

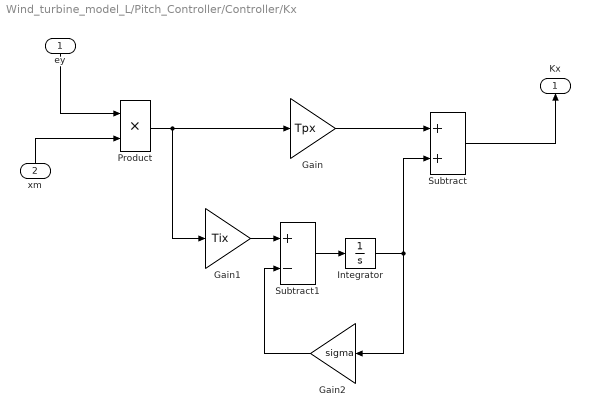
== system Wind_turbine_model_L/Pitch_Controller/Controller/Kx ==
  ey : Inport
  xm : Inport  Port=2
  Gain : Gain  Gain=Tpx
  Gain1 : Gain  Gain=Tix
  Gain2 : Gain  Gain=sigma
  Integrator : Integrator
  Product : Product
  Subtract : Sum
  Subtract1 : Sum  Inputs=+-
  Kx : Outport
  wires:
  Subtract/1 -> Kx/1
  Gain/1 -> Subtract/1
  Gain1/1 -> Subtract1/1
  Subtract1/1 -> Integrator/1
  Integrator/1 -> Gain2/1, Subtract/2
  Gain2/1 -> Subtract1/2
  Product/1 -> Gain1/1, Gain/1
  ey/1 -> Product/1
  xm/1 -> Product/2

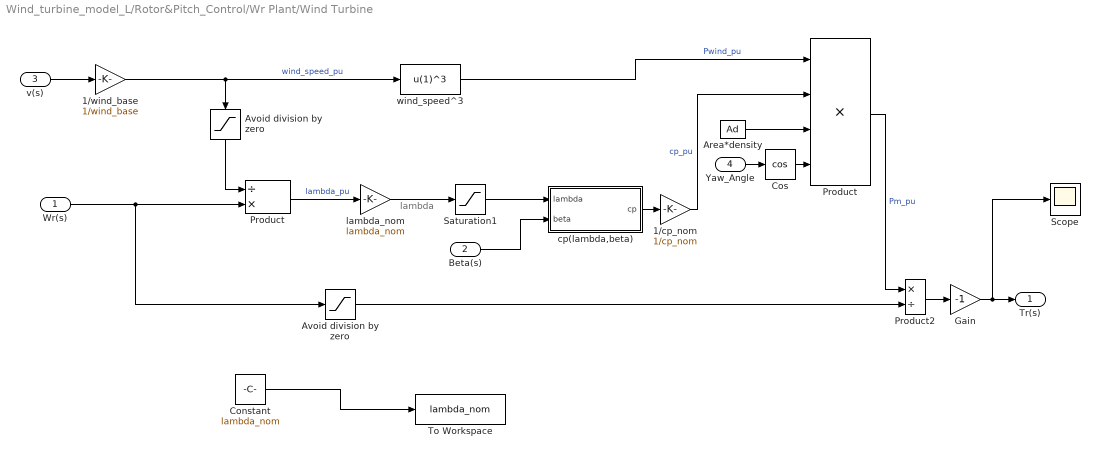
== system Wind_turbine_model_L/Rotor&Pitch_Control/Wr Plant/Wind Turbine ==
  note: lambda
  Wr(s) : Inport
  Beta(s) : Inport  Port=2
  v(s) : Inport  Port=3
  Yaw_Angle : Inport  Port=4
  1/cp_nom : Gain  Gain=1/cp_nom  SaturateOnIntegerOverflow=on  OutDataTypeStr=Inherit: Same as input  ParamDataTypeStr=Inherit: Same as input
  1/wind_base : Gain  Gain=1/wind_base  SaturateOnIntegerOverflow=on  OutDataTypeStr=Inherit: Same as input  ParamDataTypeStr=Inherit: Same as input
  Area*density : Constant  Value=Ad
  Avoid division by zero : Saturate  UpperLimit=1e6  LowerLimit=1e-6
  "Avoid division by zero " : Saturate  UpperLimit=1e6  LowerLimit=1e-6
  Constant : Constant  Value=lambda_nom
  Cos : Trigonometry  Operator=cos
  Gain : Gain  Gain=-1  SaturateOnIntegerOverflow=on  OutDataTypeStr=Inherit: Same as input  ParamDataTypeStr=Inherit: Same as input
  Product : Product  Inputs=/*  SaturateOnIntegerOverflow=on  OutDataTypeStr=Inherit: Same as first input
  "Product " : Product  Inputs=4  SaturateOnIntegerOverflow=on  OutDataTypeStr=Inherit: Same as first input
  Product2 : Product  Inputs=*/  InputSameDT=on  SaturateOnIntegerOverflow=on  OutDataTypeStr=Inherit: Same as first input
  Saturation1 : Saturate  UpperLimit=inf  LowerLimit=1e-6
  Scope : Scope
  To Workspace : ToWorkspace  VariableName=lambda_nom  SaveFormat=Timeseries  SampleTime=-1
  cp(lambda,beta) : Subsystem
  lambda_nom : Gain  Gain=lambda_nom  SaturateOnIntegerOverflow=on  OutDataTypeStr=Inherit: Same as input  ParamDataTypeStr=Inherit: Same as input
  wind_speed^3 : Fcn  Expr=u(1)^3
  Tr(s) : Outport
  wires:
  Area*density/1 -> "Product "/3
  Wr(s)/1 -> Avoid division by zero/1, Product/2
  "Avoid division by zero "/1 -> Product/1
  1/wind_base/1 -> "Avoid division by zero "/1, wind_speed^3/1  "wind_speed_pu"
  Product/1 -> lambda_nom/1  "lambda_pu"
  Saturation1/1 -> cp(lambda,beta)/1(lambda)
  1/cp_nom/1 -> "Product "/2  "cp_pu"
  lambda_nom/1 -> Saturation1/1
  "Product "/1 -> Product2/1  "Pm_pu"
  v(s)/1 -> 1/wind_base/1
  Avoid division by zero/1 -> Product2/2
  Product2/1 -> Gain/1
  wind_speed^3/1 -> "Product "/1  "Pwind_pu"
  cp(lambda,beta)/1(cp) -> 1/cp_nom/1
  Beta(s)/1 -> cp(lambda,beta)/2(beta)
  Gain/1 -> Scope/1, Tr(s)/1
  Constant/1 -> To Workspace/1
  Yaw_Angle/1 -> Cos/1
  Cos/1 -> "Product "/4

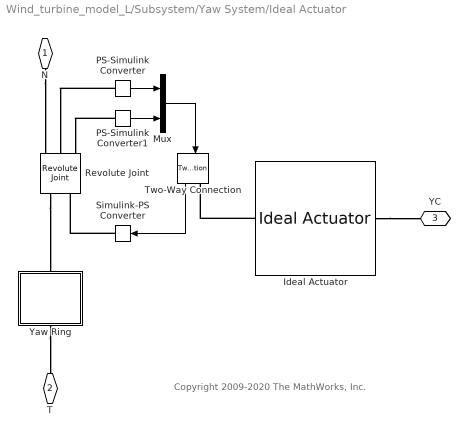
== system Wind_turbine_model_L/Subsystem/Yaw System/Ideal Actuator ==
  note: Copyright 2009-2020 The MathWorks, Inc.
  Ideal Actuator : Yaw_Actuation_Lib/Ideal Actuator  SystemSampleTime=-1  Latency=0  AutoFrameSizeCalculation=off
  Mux : Mux  Inputs=2
  PS-Simulink Converter : nesl_utility/PS-Simulink Converter  PhysicalDomain=network_engine_domain  SubClassName=ps_output  LeftPortType=input  RightPortType=output  PseudoPeriodic=off  Frequencies=[]  Unit=deg  AffineConversion=off
  PS-Simulink Converter1 : nesl_utility/PS-Simulink Converter  PhysicalDomain=network_engine_domain  SubClassName=ps_output  LeftPortType=input  RightPortType=output  PseudoPeriodic=off  Frequencies=[]  Unit=deg/s  AffineConversion=off
  Revolute Joint : sm_lib/Joints/Revolute Joint  JointMode=Normal  SenseConstraintForce=off  SenseConstraintForceX=off  SenseConstraintForceY=off  SenseConstraintForceZ=off  SenseConstraintTorque=off  SenseConstraintTorqueX=off  SenseConstraintTorqueY=off  SenseConstraintTorqueZ=off  SenseTotalForce=off  SenseTotalForceX=off  SenseTotalForceY=off  SenseTotalForceZ=off  SenseTotalTorque=off  SenseTotalTorqueX=off  SenseTotalTorqueY=off  SenseTotalTorqueZ=off  CompositeWrenchDir=FollowerOnBase  CompositeWrenchFrame=BaseFrame  EquilibriumPosition=0  EquilibriumPositionUnits=deg  SpringStiffness=0  SpringStiffnessUnits=N*m/deg  DampingCoefficient=WT_Params.Nacelle.damping  DampingCoefficientUnits=N*m/(deg/s)  TorqueActuationMode=InputTorque  MotionActuationMode=ComputedMotion  SensePosition=on  SenseVelocity=on  SenseAcceleration=off  SenseTorqueForce=off  SenseLowerLimitTorqueForce=off  SenseUpperLimitTorqueForce=off  LowerLimitSpecify=off  LowerLimitBound=-90  LowerLimitBoundUnits=deg  LowerLimitStiffness=1e4  LowerLimitStiffnessUnits=N*m/deg  LowerLimitDamping=10  LowerLimitDampingUnits=N*m/(deg/s)  LowerLimitTransitionRegionWidth=0.1  LowerLimitTransitionRegionWidthUnits=deg  UpperLimitSpecify=off  UpperLimitBound=90  UpperLimitBoundUnits=deg  UpperLimitStiffness=1e4  UpperLimitStiffnessUnits=N*m/deg  UpperLimitDamping=10  UpperLimitDampingUnits=N*m/(deg/s)  UpperLimitTransitionRegionWidth=0.1  UpperLimitTransitionRegionWidthUnits=deg  PositionTargetSpecify=off  PositionTargetPriority=High  PositionTargetValue=0  PositionTargetValueUnits=deg  VelocityTargetSpecify=off  VelocityTargetPriority=High  VelocityTargetValue=0  VelocityTargetValueUnits=deg/s
  Simulink-PS Converter : nesl_utility/Simulink-PS Converter  PhysicalDomain=network_engine_domain  SubClassName=ps_input  LeftPortType=input  RightPortType=output  PseudoPeriodic=off  Frequencies=[]  NoiseDistribution=none  NoiseParameters=[]  Unit=1  AffineConversion=off  FilteringAndDerivatives=zero  SimscapeFilterOrder=1  InputFilterTimeConstant=0.005  UdotUserProvided=[]
  Two-Way Connection : TwoWayConnection
  Yaw Ring : Subsystem
  N : PMIOPort  Side=Right
  T : PMIOPort  Port=2  Side=Left
  YC : PMIOPort  Port=3  Side=Right
  wires:
  PS-Simulink Converter/1 -> Mux/1
  Two-Way Connection/1 -> Simulink-PS Converter/1
  PS-Simulink Converter1/1 -> Mux/2
  Mux/1 -> Two-Way Connection/1
  connections:
  Ideal Actuator/RConn1 -- YC/RConn1
  Ideal Actuator/LConn1 -- Two-Way Connection/RConn1
  Revolute Joint/LConn1 -- Yaw Ring/RConn1
  PS-Simulink Converter/LConn1 -- Revolute Joint/RConn2
  N/RConn1 -- Revolute Joint/RConn1
  PS-Simulink Converter1/LConn1 -- Revolute Joint/RConn3
  Simulink-PS Converter/RConn1 -- Revolute Joint/LConn2
  Yaw Ring/LConn1 -- T/RConn1

== system Wind_turbine_model_L/Generator/Controller/Subsystem/D//Q-->alfa//beta ==
  abc : Inport
  Fcn : Fcn  Expr=2/3*(u[1]-u[2]/2-u[3]/2)
  Fcn1 : Fcn  Expr=2/3*(u[2]*(sqrt(3)/2)-u[3]*(sqrt(3)/2))
  Mux : Mux  Inputs=2
  alfa/beta : Outport
  wires:
  Mux/1 -> alfa/beta/1
  Fcn1/1 -> Mux/2
  Fcn/1 -> Mux/1
  abc/1 -> Fcn/1, Fcn1/1

== system Wind_turbine_model_L/Rotor&Pitch_Control/Wr Plant/Wind Turbine/cp(lambda,beta) ==
  lambda : Inport
  beta : Inport  Port=2
  Fcn : Fcn  Expr=1/(1/(u[1]+a7*u[2])-a8/(u[2]^3+1))
  Fcn1 : Fcn  Expr=a1*(a2/u[2]-a3*u[3]-a4)*exp(-a5/u[2])+a6*u[1]
  Mux : Mux  Inputs=2
  Mux1 : Mux  Inputs=3
  cp : Outport
  wires:
  Mux/1 -> Fcn/1
  beta/1 -> Mux/2, Mux1/3
  Mux1/1 -> Fcn1/1
  lambda/1 -> Mux/1, Mux1/1
  Fcn1/1 -> cp/1
  Fcn/1 -> Mux1/2  "lambda_i"

== system Wind_turbine_model_L/Subsystem/Yaw System/Ideal Actuator/Yaw Ring ==
  Transform Yaw Ring Center : sm_lib/Frames and Transforms/Rigid Transform  TranslationMethod=StandardAxis  TranslationStandardOffset=WT_Params.Yaw_Actuator.yaw_ring_thickness/2  TranslationLengthUnit=m  TranslationStandardAxis=+Z  TranslationCartesianOffset=[0 0 0]  TranslationROffset=0  TranslationROffsetUnits=m  TranslationZOffset=0  TranslationZOffsetUnits=m  TranslationThetaOffset=0  TranslationThetaOffsetUnits=deg  RotationMethod=None  RotationAngleUnits=deg  RotationStandardAxis=+Z  RotationAngle=0  RotationArbitraryAxis=[0 0 1]  FollAlignAxisA=+X  BaseAlignAxisA=+Y  FollAlignAxisB=+Y  BaseAlignAxisB=+Z  RotationSequenceAxes=FollowerAxes  RotationSequence=XYX  RotationSequenceAngles=[0 0 0]  RotationSequenceAnglesUnits=deg  RotationMatrix=[1 0 0; 0 1 0; 0 0 1]
  Transform Yaw Ring Top : sm_lib/Frames and Transforms/Rigid Transform  TranslationMethod=StandardAxis  TranslationStandardOffset=WT_Params.Yaw_Actuator.yaw_ring_thickness/2  TranslationLengthUnit=m  TranslationStandardAxis=+Z  TranslationCartesianOffset=[0 0 0]  TranslationROffset=0  TranslationROffsetUnits=m  TranslationZOffset=0  TranslationZOffsetUnits=m  TranslationThetaOffset=0  TranslationThetaOffsetUnits=deg  RotationMethod=None  RotationAngleUnits=deg  RotationStandardAxis=+Z  RotationAngle=0  RotationArbitraryAxis=[0 0 1]  FollAlignAxisA=+X  BaseAlignAxisA=+Y  FollAlignAxisB=+Y  BaseAlignAxisB=+Z  RotationSequenceAxes=FollowerAxes  RotationSequence=XYX  RotationSequenceAngles=[0 0 0]  RotationSequenceAnglesUnits=deg  RotationMatrix=[1 0 0; 0 1 0; 0 0 1]
  Yaw Ring : sm_lib/Body Elements/Cylindrical Solid  GraphicAmbientColor=[0.15 0.15 0.15 1.0]  BasedOnType=Density  CenterOfMass=[0 0 0]  CenterOfMassUnits=m  GraphicDiffuseColor=[1.0 1.0 0.0]  CylinderLength=WT_Params.Yaw_Actuator.yaw_ring_thickness  CylinderLengthUnits=m  CylinderRadius=WT_Params.Yaw_Actuator.yaw_ring_diameter/2  CylinderRadiusUnits=m  Density=1000  DensityUnits=kg/(m^3)  DoExposeReferenceFrame=on  GraphicEmissiveColor=[0.0 0.0 0.0 1.0]  ExportEntireGeometry=off  SerializedFrames=<Frames/>  MarkerShape=Sphere  MarkerSize=10  GraphicType=FromGeometry  InertiaType=CalculateFromGeometry  Mass=1  MassUnits=kg  MomentsOfInertia=[1 1 1]  MomentsOfInertiaUnits=kg*m^2  GraphicOpacity=1.0  ProductsOfInertia=[0 0 0]  ProductsOfInertiaUnits=kg*m^2  GraphicShininess=75  GraphicSpecularColor=[0.5 0.5 0.5 1.0]  GraphicVisPropType=SimpleVisualProperties
  N : PMIOPort  Side=Right
  T : PMIOPort  Port=2  Side=Left
  connections:
  Transform Yaw Ring Top/RConn1 -- N/RConn1
  Transform Yaw Ring Center/LConn1 -- T/RConn1
  Transform Yaw Ring Top/LConn1 -- Yaw Ring/RConn1 -- Transform Yaw Ring Center/RConn1
